simulink model "Controller_CS3"  (R2014a)
settings: Solver=ode4  StartTime=0.0  StopTime=Inf  FixedStep=0.01  MaxStep=0.01  RelTol=1e-3
undefined symbols (not defined in the file): Control, T_m_inv, T_matrix
libraries: simulink_extras x4, commnoisgen2 x1
(part 3 of 3)

== system Controller_CS3/Observers/Cont. Nonlinear Passive DP obs/Nonlinear observer/Wavefilter module1 ==
  note: Aw*eps
  note: Aw
  note: eps
  note: WAVEFILTER MODULE
      | Filters wave motions when enabled
      | in "obsdat.m". Uses design parameters determined
      | from the current seastate set in parameters.m
      | Martin Austad, 2003
  eta_error : Inport
  A(w) : Inport  Port=2
  K1(w) : Inport  Port=3
  Enable : EnablePort
  Cw : Gain  Gain=Control.VessObs.Cw  Multiplication=Matrix(K*u)  SaturateOnIntegerOverflow=on  OutDataTypeStr=Inherit: Same as input  ParamDataTypeStr=Inherit: Same as input
  Integrator : Integrator
  Product : Product  Multiplication=Matrix(*)  SaturateOnIntegerOverflow=on  OutDataTypeStr=Inherit: Same as first input
  Product1 : Product  Multiplication=Matrix(*)  SaturateOnIntegerOverflow=on  OutDataTypeStr=Inherit: Same as first input
  Sum3 : Sum  Inputs=|++  SaturateOnIntegerOverflow=on
  Wave_est : Outport
  wires:
  K1(w)/1 -> Product1/1
  A(w)/1 -> Product/1
  Product/1 -> Sum3/2
  Product1/1 -> Sum3/1
  Integrator/1 -> Product/2, Cw/1
  eta_error/1 -> Product1/2
  Cw/1 -> Wave_est/1
  Sum3/1 -> Integrator/1

== system Controller_CS3/Observers/Hybrid Nonlinear Passive DP obs/Error filter/Subsystem ==
  In1 : Inport
  gs : Inport  Port=2
  Gain : Gain  Gain=10
  Integrator : Integrator  ExternalReset=level hold
  Sum : Sum  Inputs=|+-
  Out1 : Outport
  wires:
  Sum/1 -> Gain/1
  Gain/1 -> Integrator/1
  gs/1 -> Integrator/2
  Integrator/1 -> Out1/1, Sum/2
  In1/1 -> Sum/1

== system Controller_CS3/Observers/Hybrid Nonlinear Passive DP obs/Error filter/Subsystem1 ==
  In1 : Inport
  gs : Inport  Port=2
  Gain : Gain  Gain=10
  Integrator : Integrator  ExternalReset=level hold  AbsoluteTolerance=1e-8
  Sum : Sum  Inputs=|+-
  Out1 : Outport
  wires:
  In1/1 -> Sum/1
  Gain/1 -> Integrator/1
  Sum/1 -> Gain/1
  gs/1 -> Integrator/2
  Integrator/1 -> Out1/1, Sum/2

== system Controller_CS3/Observers/Hybrid Nonlinear Passive DP obs/Error filter/Subsystem2 ==
  In1 : Inport
  gs : Inport  Port=2
  Gain : Gain  Gain=10
  Integrator : Integrator  ExternalReset=level hold
  Sum : Sum  Inputs=|+-
  Out1 : Outport
  wires:
  Sum/1 -> Gain/1
  Gain/1 -> Integrator/1
  gs/1 -> Integrator/2
  Integrator/1 -> Out1/1, Sum/2
  In1/1 -> Sum/1

== system Controller_CS3/Observers/Hybrid Nonlinear Passive DP obs/Integrator system/CT dynamics ==
  f(x,u) : Inport
  Flows : Constant
  Jumps : Constant  Value=0
  Mux : Mux  Inputs=[1 1 -1]
  dot : Outport
  wires:
  f(x,u)/1 -> Mux/3
  Mux/1 -> dot/1
  Flows/1 -> Mux/1
  Jumps/1 -> Mux/2

== system Controller_CS3/Observers/Hybrid Nonlinear Passive DP obs/Integrator system/Update logic ==
  g(x-,u) : Inport
  j- : Inport  Port=2
  t- : Inport  Port=3
  Constant : Constant
  Mux : Mux  Inputs=[1 1 -1]
  Sum : Sum  Inputs=|++
  update law : Outport
  wires:
  Mux/1 -> update law/1
  j-/1 -> Sum/1
  Sum/1 -> Mux/2
  Constant/1 -> Sum/2
  t-/1 -> Mux/1
  g(x-,u)/1 -> Mux/3

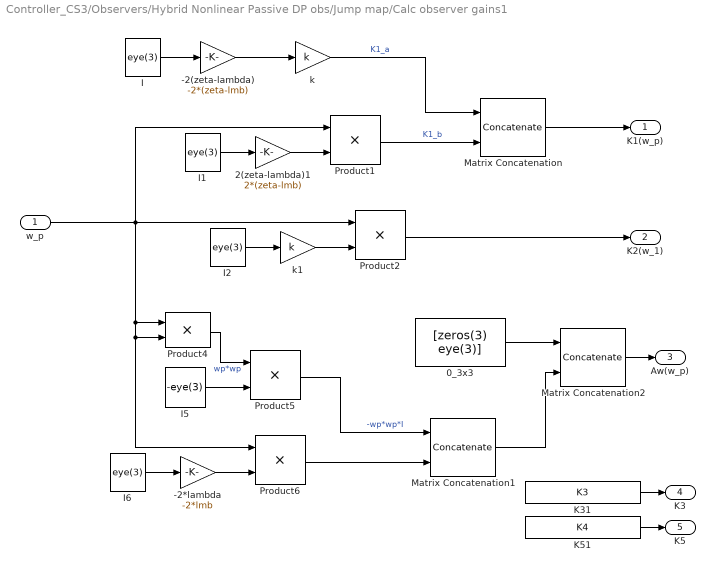
== system Controller_CS3/Observers/Hybrid Nonlinear Passive DP obs/Jump map/Calc observer gains1 ==
  w_p : Inport
  -2(zeta-lambda) : Gain  Gain=-2*(zeta-lmb)  SaturateOnIntegerOverflow=on  OutDataTypeStr=Inherit: Same as input  ParamDataTypeStr=Inherit: Same as input
  -2*lambda : Gain  Gain=-2*lmb  SaturateOnIntegerOverflow=on  OutDataTypeStr=Inherit: Same as input  ParamDataTypeStr=Inherit: Same as input
  0_3x3 : Constant  Value=[zeros(3) eye(3)]
  2(zeta-lambda)1 : Gain  Gain=2*(zeta-lmb)  SaturateOnIntegerOverflow=on  OutDataTypeStr=Inherit: Same as input  ParamDataTypeStr=Inherit: Same as input
  I{,1..2,6} (4 alike) : Constant  Value=eye(3)
  I5 : Constant  Value=-eye(3)
  K31 : Constant  Value=K3
  K51 : Constant  Value=K4
  Matrix Concatenation : Concatenate  Mode=Multidimensional array
  Matrix Concatenation1 : Concatenate  Mode=Multidimensional array  ConcatenateDimension=2
  Matrix Concatenation2 : Concatenate  Mode=Multidimensional array
  Product{1..2,4..6} (5 alike) : Product  SaturateOnIntegerOverflow=on  OutDataTypeStr=Inherit: Same as first input
  k : Gain  Gain=k  SaturateOnIntegerOverflow=on  OutDataTypeStr=Inherit: Same as input  ParamDataTypeStr=Inherit: Same as input
  k1 : Gain  Gain=k  SaturateOnIntegerOverflow=on  OutDataTypeStr=Inherit: Same as input  ParamDataTypeStr=Inherit: Same as input
  K1(w_p) : Outport
  K2(w_1) : Outport  Port=2
  Aw(w_p) : Outport  Port=3
  K3 : Outport  Port=4
  K5 : Outport  Port=5
  wires:
  Matrix Concatenation/1 -> K1(w_p)/1
  w_p/1 -> Product1/1, Product2/1, Product4/1, Product4/2, Product6/1
  I/1 -> -2(zeta-lambda)/1
  -2(zeta-lambda)/1 -> k/1
  I1/1 -> 2(zeta-lambda)1/1
  2(zeta-lambda)1/1 -> Product1/2
  Product1/1 -> Matrix Concatenation/2  "K1_b"
  I2/1 -> k1/1
  Product2/1 -> K2(w_1)/1
  k1/1 -> Product2/2
  k/1 -> Matrix Concatenation/1  "K1_a"
  Product4/1 -> Product5/1  "wp*wp"
  I5/1 -> Product5/2
  Product5/1 -> Matrix Concatenation1/1  "-wp*wp*I"
  I6/1 -> -2*lambda/1
  -2*lambda/1 -> Product6/2
  Product6/1 -> Matrix Concatenation1/2
  Matrix Concatenation1/1 -> Matrix Concatenation2/2
  0_3x3/1 -> Matrix Concatenation2/1
  Matrix Concatenation2/1 -> Aw(w_p)/1
  K31/1 -> K3/1
  K51/1 -> K5/1

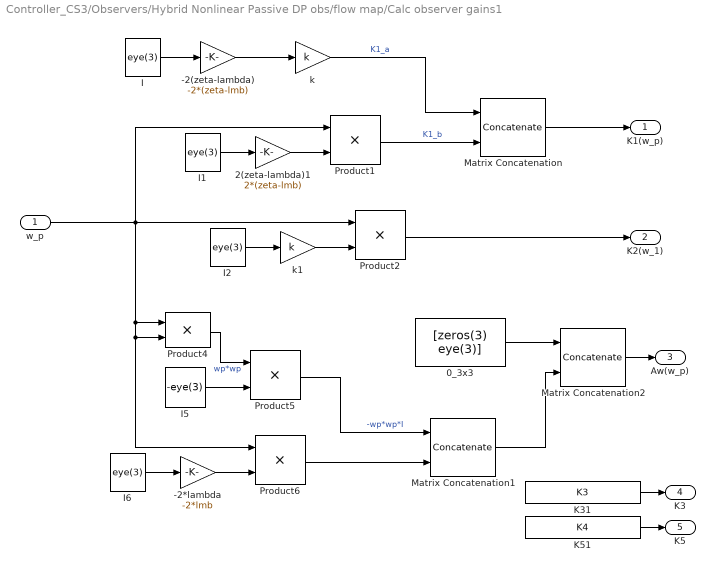
== system Controller_CS3/Observers/Hybrid Nonlinear Passive DP obs/flow map/Calc observer gains1 ==
  w_p : Inport
  -2(zeta-lambda) : Gain  Gain=-2*(zeta-lmb)  SaturateOnIntegerOverflow=on  OutDataTypeStr=Inherit: Same as input  ParamDataTypeStr=Inherit: Same as input
  -2*lambda : Gain  Gain=-2*lmb  SaturateOnIntegerOverflow=on  OutDataTypeStr=Inherit: Same as input  ParamDataTypeStr=Inherit: Same as input
  0_3x3 : Constant  Value=[zeros(3) eye(3)]
  2(zeta-lambda)1 : Gain  Gain=2*(zeta-lmb)  SaturateOnIntegerOverflow=on  OutDataTypeStr=Inherit: Same as input  ParamDataTypeStr=Inherit: Same as input
  I{,1..2,6} (4 alike) : Constant  Value=eye(3)
  I5 : Constant  Value=-eye(3)
  K31 : Constant  Value=K3
  K51 : Constant  Value=K4
  Matrix Concatenation : Concatenate  Mode=Multidimensional array
  Matrix Concatenation1 : Concatenate  Mode=Multidimensional array  ConcatenateDimension=2
  Matrix Concatenation2 : Concatenate  Mode=Multidimensional array
  Product{1..2,4..6} (5 alike) : Product  SaturateOnIntegerOverflow=on  OutDataTypeStr=Inherit: Same as first input
  k : Gain  Gain=k  SaturateOnIntegerOverflow=on  OutDataTypeStr=Inherit: Same as input  ParamDataTypeStr=Inherit: Same as input
  k1 : Gain  Gain=k  SaturateOnIntegerOverflow=on  OutDataTypeStr=Inherit: Same as input  ParamDataTypeStr=Inherit: Same as input
  K1(w_p) : Outport
  K2(w_1) : Outport  Port=2
  Aw(w_p) : Outport  Port=3
  K3 : Outport  Port=4
  K5 : Outport  Port=5
  wires:
  K51/1 -> K5/1
  K31/1 -> K3/1
  Matrix Concatenation2/1 -> Aw(w_p)/1
  0_3x3/1 -> Matrix Concatenation2/1
  Matrix Concatenation1/1 -> Matrix Concatenation2/2
  Product6/1 -> Matrix Concatenation1/2
  -2*lambda/1 -> Product6/2
  I6/1 -> -2*lambda/1
  Product5/1 -> Matrix Concatenation1/1  "-wp*wp*I"
  I5/1 -> Product5/2
  Product4/1 -> Product5/1  "wp*wp"
  k/1 -> Matrix Concatenation/1  "K1_a"
  k1/1 -> Product2/2
  Product2/1 -> K2(w_1)/1
  I2/1 -> k1/1
  Product1/1 -> Matrix Concatenation/2  "K1_b"
  2(zeta-lambda)1/1 -> Product1/2
  I1/1 -> 2(zeta-lambda)1/1
  -2(zeta-lambda)/1 -> k/1
  I/1 -> -2(zeta-lambda)/1
  w_p/1 -> Product6/1, Product4/2, Product4/1, Product2/1, Product1/1
  Matrix Concatenation/1 -> K1(w_p)/1

== matlab function Controller_CS3/Thruster system comp/signal check thr 1 ==
  data: u input; rps output
function rps = fcn(u)
%#codegen

if abs(u) > 100000
  u = 0;
elseif abs(u) < 200 && abs(u) > 100
  u = 200;
elseif abs(u) <= 100
  u = 0;
end

if abs(u) < 100000 && abs(u) >= 200
   rps = (10000/u); 
else
   rps = 0; 
end

== matlab function Controller_CS3/u 2 rps/MATLAB Function ==
  data: u input; rps output; Kt_p input; Kt_n input; d input; rho input
function rps = fcn(u,Kt_p,Kt_n,d,rho)
%#codegen

if u >= 0
   rps = sqrt(u/(Kt_p*d^4*rho)); 
else
   rps = -sqrt(abs(u)/(Kt_n*d^4*rho)); 
end

== matlab function Controller_CS3/Observers/Hybrid Nonlinear Passive DP obs/Jump map/jump map g ==
  data: x input; y input; K1 input; K2 input; Aw input; K3 input; K5 input; M_inv input; D input; e input; g_max input; gs input; wave_filter_onoff input; x_plus output double
function x_plus  = f(x,y,K1,K2,Aw,K3,K5,M_inv,D,e,g_max,gs,wave_filter_onoff) 

%%%%%%%%%%%%%%%%%%%%%%%%%%%%%%%%%%%%%%%%%%%%%%%%%%%%%%%%%%%%%%%%%%%%%%%%%%%
% Matlab Function  Author: Ricardo Sanfelice 
% (Revised by Giampiero Campa)
% (Revised by Pablo Nanez)
%
% Project: Simulation of a hybrid system (Bouncing Ball)
%
% Name: f.m
%
% Description: Flow map
%
% Version: 1.0
% Required files: - 
%%%%%%%%%%%%%%%%%%%%%%%%%%%%%%%%%%%%%%%%%%%%%%%%%%%%%%%%%%%%%%%%%%%%%%%%%%%


% flow map: xdot=f(x,u);

R = [cos(y(3)) -sin(y(3)) 0;
    sin(y(3)) cos(y(3)) 0;
    0 0 1];


if wave_filter_onoff
    
    A = [Aw zeros(6,9);
        zeros(3,9) R zeros(3);
        zeros(3,9) -M_inv*D M_inv*(R');
        zeros(3,15)];

    L = [K1;
        K2;
        M_inv*(R')*K5;
        K3];

    C = [zeros(3) eye(3) eye(3) zeros(3) zeros(3)];

    H = A-L*C;

    x_err = -inv(H)*[zeros(3,12) eye(3)]'*(diag(gs)*diag(sign(e))*g_max);

    x_plus = x + x_err;
    
else
    
    A = [zeros(6,15);
        zeros(3,9) R zeros(3);
        zeros(3,9) -M_inv*D M_inv*(R');
        zeros(3,15)];
    
    L = [zeros(6,3);
        K2;
        M_inv*(R')*K5;
        K3];

    C = [zeros(3) zeros(3) eye(3) zeros(3) zeros(3)];

    H = A(7:15,7:15)-L(7:15,:)*C(:,7:15);

    x_err_0 = -inv(H)*[zeros(3,6) eye(3)]'*(diag(gs)*diag(sign(e))*g_max);
    
    x_err = [zeros(6,1);
            x_err_0];
    
    x_plus = x + x_err;
end

== matlab function Controller_CS3/Observers/Hybrid Nonlinear Passive DP obs/flow map/flow map f ==
  data: x input; y input; tau input; xdot output double; K1 input; K2 input; Aw input; K3 input; K5 input; M_inv input; D input; wave_filter_onoff input
function xdot  = f(x,y,tau,K1,K2,Aw,K3,K5,M_inv,D,wave_filter_onoff) 

%%%%%%%%%%%%%%%%%%%%%%%%%%%%%%%%%%%%%%%%%%%%%%%%%%%%%%%%%%%%%%%%%%%%%%%%%%%
% Matlab Function  Author: Ricardo Sanfelice 
% (Revised by Giampiero Campa)
% (Revised by Pablo Nanez)
%
% Project: Simulation of a hybrid system (Bouncing Ball)
%
% Name: f.m
%
% Description: Flow map
%
% Version: 1.0
% Required files: - 
%%%%%%%%%%%%%%%%%%%%%%%%%%%%%%%%%%%%%%%%%%%%%%%%%%%%%%%%%%%%%%%%%%%%%%%%%%%


% flow map: xdot=f(x,u);

R = [cos(y(3)) -sin(y(3)) 0;
    sin(y(3)) cos(y(3)) 0;
    0 0 1];

if wave_filter_onoff
    
    A = [Aw zeros(6,9);
        zeros(3,9) R zeros(3);
        zeros(3,9) -M_inv*D M_inv*(R');
        zeros(3,15)];

    B = [zeros(9,3);
        M_inv;
        zeros(3)];

    L = [K1;
        K2;
        M_inv*(R')*K5;
        K3];

    C = [zeros(3) eye(3) eye(3) zeros(3) zeros(3)];

    xdot = A*x + B*tau + L*(y-C*x);
else
    
    A = [zeros(6,15);
        zeros(3,9) R zeros(3);
        zeros(3,9) -M_inv*D M_inv*(R');
        zeros(3,15)];

    B = [zeros(9,3);
        M_inv;
        zeros(3)];

    L = [zeros(6,3);
        K2;
        M_inv*(R')*K5;
        K3];

    C = [zeros(3) zeros(3) eye(3) zeros(3) zeros(3)];

    xdot = A*x + B*tau + L*(y-C*x);
end

== matlab function Controller_CS3/Observers/Hybrid Nonlinear Passive DP obs/jump set D ==
  data: v output double; gs output; e input; epsilon input; t input
function [v,gs]  = D(e,epsilon,t) 

%%%%%%%%%%%%%%%%%%%%%%%%%%%%%%%%%%%%%%%%%%%%%%%%%%%%%%%%%%%%%%%%%%%%%%%%%%%
% Matlab Function  Author: Ricardo Sanfelice 
% (Revised by Giampiero Campa)
% (Revised by Pablo Nanez)
%
% Project: Simulation of a hybrid system (Bouncing ball)
%
% Name: D.m
%
% Description: Jump set
%
% Version: 1.0
% Required files: - 
%%%%%%%%%%%%%%%%%%%%%%%%%%%%%%%%%%%%%%%%%%%%%%%%%%%%%%%%%%%%%%%%%%%%%%%%%%%
% 
% if (x(1) <= u(1)) && (x(2) <= 0)  % jump condition
%     v = 1;  % report jump
% else
%     v = 0;   % do not report jump
% end

v = 0;
gs = [0 0 0]';

if abs(e(1)) > epsilon(1) && t > 3
    v = 1;
    gs(1) = 1;
end

if abs(e(2)) > epsilon(2) && t > 3
    v = 1;
    gs(2) = 1;
end

if abs(e(3)) > epsilon(3) && t > 3
    v = 1;
    gs(3) = 1;
end

== matlab function Controller_CS3/Thruster system comp/signal check thr 2 ==
  data: u input; rps output
function rps = fcn(u)
%#codegen

if abs(u) > 100000
  u = 0;
elseif abs(u) < 200 && abs(u) > 100
  u = 200;
elseif abs(u) <= 100
  u = 0;
end

if abs(u) < 100000 && abs(u) >= 200
   rps = (10000/u); 
else
   rps = 0; 
end

== matlab function Controller_CS3/Control law/Rst logics/MATLAB Function ==
  data: rst_in input; eta_hat input; eta_d_in input; rst output; eta_d output; eta_d_prev input
function [rst, eta_d] = fcn(rst_in,eta_hat,eta_d_in,eta_d_prev)
%#codegen

persistent eta_d_m;
persistent rst_m;

if isempty(rst_m)
   rst_m = 0; 
end

if isempty(eta_d_m) || rst_m == 0 && rst_in == 1
   eta_d_m = eta_hat;
end

rst_m = rst_in;
rst = rst_m;

if (eta_d_in(1) ~= eta_d_prev(1) || eta_d_in(2) ~= eta_d_prev(2) || eta_d_in(3) ~= eta_d_prev(3)) && rst == 1
   rst = 0;
   eta_d_m = eta_d_in;
end

eta_d = eta_d_m;

== matlab function Controller_CS3/u 2 rps1/MATLAB Function ==
  data: u input; rps output; Kt_p input; Kt_n input; d input; rho input
function rps = fcn(u,Kt_p,Kt_n,d,rho)
%#codegen

if u >= 0
   rps = sqrt(u/(Kt_p*d^4*rho)); 
else
   rps = -sqrt(abs(u)/(Kt_n*d^4*rho)); 
end

== matlab function Controller_CS3/u 2 rps2/MATLAB Function ==
  data: u input; rps output; Kt_p input; Kt_n input; d input; rho input
function rps = fcn(u,Kt_p,Kt_n,d,rho)
%#codegen

if u >= 0
   rps = sqrt(u/(Kt_p*d^4*rho)); 
else
   rps = -sqrt(abs(u)/(Kt_n*d^4*rho)); 
end

== matlab function Controller_CS3/Thruster system comp/signal check thr 3 ==
  data: u input; rps output
function rps = fcn(u)
%#codegen

if abs(u) > 100000
  u = 0;
elseif abs(u) < 200 && abs(u) > 100
  u = 200;
elseif abs(u) <= 100
  u = 0;
end

if abs(u) < 100000 && abs(u) >= 200
   rps = (10000/u); 
else
   rps = 0; 
end

== matlab function Controller_CS3/Generalized force computation/MATLAB Function ==
  data: u output; rps input; Kt_p input; Kt_n input; d input; rho input
function u = fcn(rps,Kt_p,Kt_n,d,rho)
%#codegen

if rps >= 0
   u = Kt_p*rps^2*d^4*rho; 
else
   u = -Kt_n*rps^2*d^4*rho; 
end

== matlab function Controller_CS3/Generalized force computation/MATLAB Function1 ==
  data: u output; rps input; Kt_p input; Kt_n input; d input; rho input
function u = fcn(rps,Kt_p,Kt_n,d,rho)
%#codegen

if rps >= 0
   u = Kt_p*rps^2*d^4*rho; 
else
   u = -Kt_n*rps^2*d^4*rho; 
end

== matlab function Controller_CS3/Generalized force computation/MATLAB Function2 ==
  data: u output; rps input; Kt_p input; Kt_n input; d input; rho input
function u = fcn(rps,Kt_p,Kt_n,d,rho)
%#codegen

if rps >= 0
   u = Kt_p*rps^2*d^4*rho; 
else
   u = -Kt_n*rps^2*d^4*rho; 
end
